simulink model "linear_ss_control_reg_obs"  (R2019b)
settings: Solver=ode45  StartTime=0.0  StopTime=1500  MaxStep=0.01  RelTol=1e-8
settings Model: Creator=Hector  LastModifiedBy=Hector

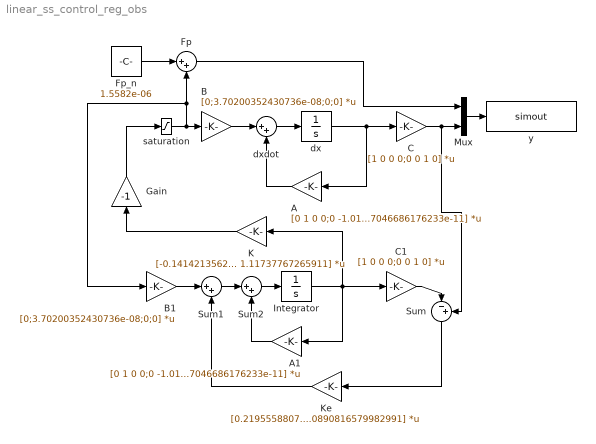
== system linear_ss_control_reg_obs ==
  A : Gain  Gain=[0 1 0 0;0 -1.01409337235247e-10 -1.70834505909243e-20 -3.36920663455173e-10;0 0 0 1;0 15365.0510962495 3.88260240702825e-06 -5.07046686176233e-11]  Multiplication=Matrix(K*u)
  A1 : Gain  Gain=[0 1 0 0;0 -1.01409337235247e-10 -1.70834505909243e-20 -3.36920663455173e-10;0 0 0 1;0 15365.0510962495 3.88260240702825e-06 -5.07046686176233e-11]  Multiplication=Matrix(K*u)
  B : Gain  Gain=[0;3.70200352430736e-08;0;0]  Multiplication=Matrix(K*u)
  B1 : Gain  Gain=[0;3.70200352430736e-08;0;0]  Multiplication=Matrix(K*u)
  C : Gain  Gain=[1 0 0 0;0 0 1 0]  Multiplication=Matrix(K*u)
  C1 : Gain  Gain=[1 0 0 0;0 0 1 0]  Multiplication=Matrix(K*u)
  Fp : Sum  Inputs=|++
  Fp_n : Constant  Value=1.5582e-06
  Gain : Gain  Gain=-1
  Integrator : Integrator  InitialCondition=[0, 0, -1*10^-3, 0].'
  K : Gain  Gain=[-0.141421356249834 963078.733398081 0.010243364845765 1.11737767265911]  Multiplication=Matrix(K*u)
  Ke : Gain  Gain=[0.219555880769803 -6.20274847519216e-06;0.0115827344660038 -5.53693888523524e-07;13913.3056289779 0.159444119063664;3243.30558114425 -0.0890816579982991]  Multiplication=Matrix(K*u)
  Mux : Mux  Inputs=2
  Sum : Sum  Inputs=|-+
  Sum1 : Sum  Inputs=|++
  Sum2 : Sum  Inputs=|++
  dx : Integrator  InitialCondition=[0, 0, -1*10^-3, 0].'
  dxdot : Sum  Inputs=|++
  saturation : Saturate  UpperLimit=1.8442e-05  LowerLimit=-1.5582e-06
  y : ToWorkspace  VariableName=simout  SaveFormat=Timeseries  SampleTime=-1
  wires:
  dxdot/1 -> dx/1
  A/1 -> dxdot/2
  dx/1 -> C/1, A/1
  B/1 -> dxdot/1
  K/1 -> Gain/1
  Fp_n/1 -> Fp/1
  Gain/1 -> saturation/1
  Mux/1 -> y/1
  C/1 -> Sum/2, Mux/2
  Fp/1 -> Mux/1
  saturation/1 -> B1/1, Fp/2, B/1
  C1/1 -> Sum/1
  Sum/1 -> Ke/1
  Sum1/1 -> Sum2/1
  A1/1 -> Sum2/2
  Sum2/1 -> Integrator/1
  Integrator/1 -> C1/1, K/1, A1/1
  B1/1 -> Sum1/1
  Ke/1 -> Sum1/2
